simulink model "feedback_control"  (R2016a)
settings: Solver=FixedStepDiscrete  StartTime=0.0  StopTime=10.0  FixedStep=T_sample_control  RelTol=1e-3
undefined symbols (not defined in the file): T_sample_control
settings Model: ModifiedByFormat=The MathWorks Inc.  Creator=The MathWorks, Inc.  LastModifiedBy=The MathWorks Inc.
settings DataIOCC: SaveFormat=Array
settings OptimizationCC: DefaultParameterBehavior=Inlined  InlineInvariantSignals=on  PassReuseOutputArgsAs=Individual arguments  ExpressionDepthLimit=2147483647  ZeroExternalMemoryAtStartup=off  ZeroInternalMemoryAtStartup=off  EfficientFloat2IntCast=on  OptimizeModelRefInitCode=on  LifeSpan=1
settings DebuggingCC: SolverPrmCheckMsg=warning  FcnCallInpInsideContextMsg=EnableAllAsWarning  UniqueDataStoreMsg=error  AssertControl=DisableAll  AllowSymbolicDim=off  StateNameClashWarn=warning  StrictBusMsg=ErrorOnBusTreatedAsVector
settings HardwareCC: ProdBitPerPointer=32  ProdLargestAtomicInteger=Long  ProdLargestAtomicFloat=Double  ProdWordSize=32  ProdHWDeviceType=ARM Compatible->ARM Cortex
settings ModelReferenceCC: PropagateSignalLabelsOutOfModel=off
settings RTWCC: SystemTargetFile=ert.tlc  GenCodeOnly=on  TemplateMakefile=ert_default_tmf  GenerateReport=on  IncludeHyperlinkInReport=on  GenerateTraceInfo=on  GenerateTraceReport=on  GenerateTraceReportSl=on  GenerateTraceReportSf=on  GenerateTraceReportEml=on  GenerateCodeMetricsReport=on
settings CodeAppCC: IgnoreCustomStorageClasses=off  IgnoreTestpoints=on  CustomSymbolStrType=$N$R$M  InternalIdentifier=Classic
settings ERTTargetCC: GenerateSampleERTMain=on  MultiInstanceERTCode=on  CodeInterfacePackaging=Reusable function  ParenthesesLevel=Maximum  InlinedParameterPlacement=NonHierarchical  ERTCustomFileTemplate=example_file_process.tlc  ERTFilePackagingFormat=Compact  ConvertIfToSwitch=off  SuppressUnreachableDefaultCases=off
settings ConfigComp: CovModelRefEnable=Off  CovSFcnEnable=off

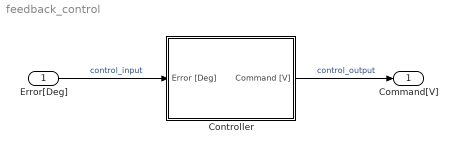
== system feedback_control ==
  Error[Deg] : Inport  OutDataTypeStr=double  PortDimensions=1  SampleTime=T_sample_control
  Controller : Subsystem
  Command[V] : Outport  OutDataTypeStr=double  PortDimensions=1  SampleTime=T_sample_control
  wires:
  Error[Deg]/1 -> Controller/1(Error [Deg])  "control_input"
  Controller/1(Command [V]) -> Command[V]/1  "control_output"

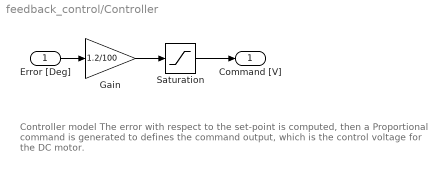
== system feedback_control/Controller ==
  note: Controller model
      | The error with respect to the set-point is computed, then a Proportional command
      | is generated to defines the command output, which is the control voltage for the DC motor.
  Error [Deg] : Inport
  Gain : Gain  Gain=1.2/100
  Saturation : Saturate  UpperLimit=1  LowerLimit=-1
  Command [V] : Outport
  wires:
  Gain/1 -> Saturation/1
  Error [Deg]/1 -> Gain/1
  Saturation/1 -> Command [V]/1
